simulink model "BatterySimulationSinusoidalCC"  (R2018b)
settings: Solver=VariableStepAuto  StartTime=0.0  StopTime=0.5  RelTol=1e-3
settings Model: Creator=GRosp  LastModifiedBy=GRosp

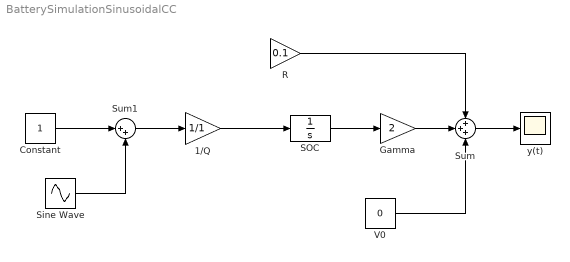
== system BatterySimulationSinusoidalCC ==
  1/Q : Gain  Gain=1/1
  Constant : Constant
  "Gamma " : Gain  Gain=2
  R : Gain  Gain=0.1
  SOC : Integrator
  Sine Wave : Sin  Amplitude=0.2  Frequency=0.01  SampleTime=0.01
  Sum : Sum  Inputs=+++
  Sum1 : Sum  Inputs=|++
  V0 : Constant  Value=0
  "y(t) " : Scope
  wires:
  1/Q/1 -> SOC/1
  SOC/1 -> "Gamma "/1
  R/1 -> Sum/1
  "Gamma "/1 -> Sum/2
  V0/1 -> Sum/3
  Sum/1 -> "y(t) "/1
  Constant/1 -> Sum1/1
  Sine Wave/1 -> Sum1/2
  Sum1/1 -> 1/Q/1
